simulink model "honors_drone"  (R2017a)
settings: Solver=FixedStepAuto  StartTime=0.0  StopTime=10.0  FixedStep=0.1  RelTol=1e-3
settings Model: Creator=s154530  LastModifiedBy=s166315
settings DataIOCC: SaveFormat=Array

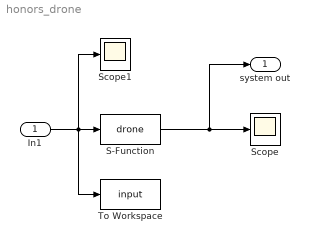
== system honors_drone ==
  In1 : Inport
  S-Function : S-Function  FunctionName=drone  Parameters=x0, m, g, Ix, Iy, Iz  SFunctionDeploymentMode=off  EnableBusSupport=off
  Scope : Scope
  Scope1 : Scope
  To Workspace : ToWorkspace  VariableName=input  SaveFormat=Timeseries  SampleTime=-1
      settings: MaxDataPoints=Inf
  system out : Outport
  wires:
  S-Function/1 -> system out/1, Scope/1
  In1/1 -> To Workspace/1, Scope1/1, S-Function/1
